simulink model "gm_wlanhdlTimeAndFrequencySynchronization"  (R2025a)
settings: Solver=FixedStepDiscrete  StartTime=0.0  StopTime=stopTime  RelTol=1e-3
InitFcn:
  | wlanFrontEndInit;
undefined symbols (not defined in the file or in its folder): a, b, c, Hd, wlanConfig
libraries: simulink x95, hdlsllib x16, hdlmdlgenlib x12, dspsrcs4 x3, dspsigops x3, dsphdlsigops2 x2, dsphdlfiltering2 x2
(part 5 of 11)

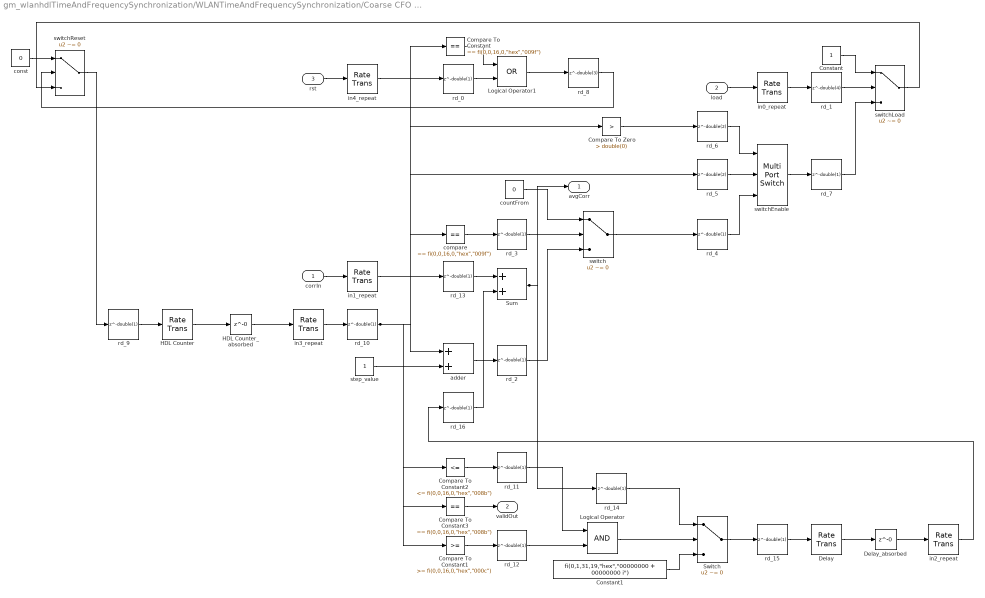
== system gm_wlanhdlTimeAndFrequencySynchronization/WLANTimeAndFrequencySynchronization/Coarse CFO Estimation and Correction/Coarse CFO Estimation/Averager ==
  corrIn : Inport  OutDataTypeStr=fixdt(1, 31, 19)  PortDimensions=1  SampleTime=5e-08
      settings: SignalType=complex
  load : Inport  Port=2  OutDataTypeStr=boolean  PortDimensions=1  SampleTime=5e-08
  rst : Inport  Port=3  OutDataTypeStr=boolean  PortDimensions=1  SampleTime=5e-08
  Compare To Constant : simulink/Logic and Bit Operations/Compare To Constant  relop===  const="fi(0,0,16,0,\"hex\",\"009f\")"  OutDataTypeStr=boolean
  Compare To Constant1 : simulink/Logic and Bit Operations/Compare To Constant  relop=>=  const="fi(0,0,16,0,\"hex\",\"000c\")"  OutDataTypeStr=boolean
  Compare To Constant2 : simulink/Logic and Bit Operations/Compare To Constant  relop=<=  const="fi(0,0,16,0,\"hex\",\"008b\")"  OutDataTypeStr=boolean
  Compare To Constant3 : simulink/Logic and Bit Operations/Compare To Constant  relop===  const="fi(0,0,16,0,\"hex\",\"008b\")"  OutDataTypeStr=boolean
  Compare To Zero : simulink/Logic and Bit Operations/Compare To Constant  relop=>  const=double(0)  OutDataTypeStr=boolean
  Constant : Constant  OutDataTypeStr=uint16  SampleTime=6.25e-09
  Constant1 : Constant  Value="fi(0,1,31,19,\"hex\",\"00000000 + 00000000 i\")"  OutDataTypeStr=fixdt(1, 31, 19)  SampleTime=6.25e-09
  Delay : RateTransition  InitialCondition=double(0)  OutPortSampleTimeOpt=Multiple of input port sample time  OutPortSampleTimeMultiple=8
  Delay_absorbed : Delay  DelayLength=0
  HDL Counter : RateTransition  InitialCondition=double(0)  OutPortSampleTimeOpt=Multiple of input port sample time  OutPortSampleTimeMultiple=8
  HDL Counter_absorbed : Delay  DelayLength=0
  Logical Operator : Logic  AllPortsSameDT=off  OutDataTypeStr=boolean  SampleTime=6.25e-09
  Logical Operator1 : Logic  Operator=OR  AllPortsSameDT=off  OutDataTypeStr=boolean  SampleTime=6.25e-09
  Sum : Sum  OutDataTypeStr=fixdt(1, 31, 19)  AccumDataTypeStr=fixdt(1, 32, 19)  SampleTime=6.25e-09
  Switch : Switch  Criteria=u2 ~= 0  Threshold="fi(0,0,1,0,\"hex\",\"0\")"  OutDataTypeStr=fixdt(1, 31, 19)  SampleTime=6.25e-09  SaturateOnIntegerOverflow=off  InputSameDT=off
  adder : Sum  OutDataTypeStr=uint16  AccumDataTypeStr=uint16  SampleTime=6.25e-09
  compare : simulink/Logic and Bit Operations/Compare To Constant  relop===  const="fi(0,0,16,0,\"hex\",\"009f\")"  OutDataTypeStr=boolean
  const : Constant  Value=0  VectorParams1D=off  OutDataTypeStr=uint16  SampleTime=6.25e-09
  countFrom : Constant  Value=0  VectorParams1D=off  OutDataTypeStr=uint16  SampleTime=6.25e-09
  in0_repeat : RateTransition  Integrity=off  Deterministic=off  OutPortSampleTimeOpt=Multiple of input port sample time  OutPortSampleTimeMultiple=1/8
  in1_repeat : RateTransition  Integrity=off  Deterministic=off  OutPortSampleTimeOpt=Multiple of input port sample time  OutPortSampleTimeMultiple=1/8
  in2_repeat : RateTransition  Integrity=off  Deterministic=off  OutPortSampleTimeOpt=Multiple of input port sample time  OutPortSampleTimeMultiple=1/8
  in3_repeat : RateTransition  Integrity=off  Deterministic=off  OutPortSampleTimeOpt=Multiple of input port sample time  OutPortSampleTimeMultiple=1/8
  in4_repeat : RateTransition  Integrity=off  Deterministic=off  OutPortSampleTimeOpt=Multiple of input port sample time  OutPortSampleTimeMultiple=1/8
  rd_{0,2..4,7,9..16} (13 alike) : Delay  DelayLength=double(1)  InitialCondition=0  SampleTime=6.25e-09
  rd_1 : Delay  DelayLength=double(4)  InitialCondition=0  SampleTime=6.25e-09
  rd_5 : Delay  DelayLength=double(2)  InitialCondition=0  SampleTime=6.25e-09
  rd_6 : Delay  DelayLength=double(2)  InitialCondition=0  SampleTime=6.25e-09
  rd_8 : Delay  DelayLength=double(3)  InitialCondition=0  SampleTime=6.25e-09
  step_value : Constant  VectorParams1D=off  OutDataTypeStr=uint16  SampleTime=6.25e-09
  switch : Switch  Criteria=u2 ~= 0  Threshold="fi(0,0,1,0,\"hex\",\"0\")"  OutDataTypeStr=uint16  SampleTime=6.25e-09  SaturateOnIntegerOverflow=off  InputSameDT=off
  switchEnable : MultiPortSwitch  DataPortOrder=Zero-based contiguous  Inputs=2  DiagnosticForDefault=None  zeroidx=on  OutDataTypeStr=uint16  SampleTime=6.25e-09  SaturateOnIntegerOverflow=off  InputSameDT=off
  switchLoad : Switch  Criteria=u2 ~= 0  Threshold="fi(0,0,1,0,\"hex\",\"0\")"  OutDataTypeStr=uint16  SampleTime=6.25e-09  SaturateOnIntegerOverflow=off  InputSameDT=off
  switchReset : Switch  Criteria=u2 ~= 0  Threshold="fi(0,0,1,0,\"hex\",\"0\")"  OutDataTypeStr=uint16  SampleTime=6.25e-09  SaturateOnIntegerOverflow=off  InputSameDT=off
  avgCorr : Outport  SampleTime=6.25e-09
  validOut : Outport  Port=2  SampleTime=6.25e-09
  wires:
  in2_repeat/1 -> rd_16/1
  Delay/1 -> Delay_absorbed/1
  rd_7/1 -> switchLoad/3
  rd_1/1 -> switchLoad/2
  Constant/1 -> switchLoad/1
  in0_repeat/1 -> rd_1/1
  Switch/1 -> rd_15/1
  rd_4/1 -> switchEnable/3
  rd_5/1 -> switchEnable/2
  load/1 -> in0_repeat/1
  Constant1/1 -> Switch/3
  rd_15/1 -> Delay/1
  rd_6/1 -> switchEnable/1
  Logical Operator/1 -> Switch/2
  switch/1 -> rd_4/1
  Compare To Zero/1 -> rd_6/1
  step_value/1 -> adder/2
  rd_3/1 -> switch/2
  rd_13/1 -> Sum/1
  rd_10/1 -> Compare To Constant3/1, Compare To Constant2/1, adder/1, compare/1, Compare To Constant/1, Compare To Constant1/1, rd_5/1, Compare To Zero/1
  Logical Operator1/1 -> rd_8/1
  Delay_absorbed/1 -> in2_repeat/1
  in3_repeat/1 -> rd_10/1
  adder/1 -> rd_2/1
  in1_repeat/1 -> rd_13/1
  HDL Counter/1 -> HDL Counter_absorbed/1
  rst/1 -> in4_repeat/1
  Compare To Constant2/1 -> rd_11/1
  rd_9/1 -> HDL Counter/1
  HDL Counter_absorbed/1 -> in3_repeat/1
  Sum/1 -> avgCorr/1, rd_14/1
  switchReset/1 -> rd_9/1
  Compare To Constant/1 -> Logical Operator1/1
  corrIn/1 -> in1_repeat/1
  const/1 -> switchReset/1
  compare/1 -> rd_3/1
  rd_16/1 -> Sum/2
  Compare To Constant1/1 -> rd_12/1
  Compare To Constant3/1 -> validOut/1
  switchEnable/1 -> rd_7/1
  rd_14/1 -> Switch/1
  countFrom/1 -> switch/1
  rd_0/1 -> Logical Operator1/2
  rd_2/1 -> switch/3
  switchLoad/1 -> switchReset/3
  rd_11/1 -> Logical Operator/1
  rd_12/1 -> Logical Operator/2
  in4_repeat/1 -> rd_0/1
  rd_8/1 -> switchReset/2

== system gm_wlanhdlTimeAndFrequencySynchronization/WLANTimeAndFrequencySynchronization/Coarse CFO Estimation and Correction/Coarse CFO Estimation/Correlator ==
  dataIn : Inport  OutDataTypeStr=fixdt(1, 16, 12)  PortDimensions=1  SampleTime=5e-08
      settings: SignalType=complex
  lstf_start : Inport  Port=2  OutDataTypeStr=boolean  PortDimensions=1  SampleTime=6.25e-09
  Data Type Conversion : DataTypeConversion  OutDataTypeStr=fixdt(1, 31, 19)  SampleTime=6.25e-09  SaturateOnIntegerOverflow=off  RndMeth=Floor
  Delay1 : Delay  DelayLength=double(2)  InitialCondition=0  SampleTime=5e-08
  Delay2 : Delay  DelayLength=double(16)  InitialCondition=0  SampleTime=5e-08
  Delay3 : Delay  DelayLength=double(2)  InitialCondition=0  SampleTime=5e-08
  Delay4 : Delay  DelayLength=double(15)  InitialCondition=0  SampleTime=5e-08
  Delay41 : RateTransition  InitialCondition=double(0)  OutPortSampleTimeOpt=Multiple of input port sample time  OutPortSampleTimeMultiple=8
  Delay5 : Delay  DelayLength=double(2)  InitialCondition=0  SampleTime=5e-08
  HwModeRegister{,1..9} (10 alike) : Delay  DelayLength=double(1)  InitialCondition=0  SampleTime=6.25e-09
  MultiplyAdd : hdlsllib/HDL Operations/Multiply-Add  Function=c-(a.*b)  datatype=fixdt(1, 33, 24)  RndMeth=Round  DoSatur=off  FMA=off
  MultiplyAdd1 : hdlsllib/HDL Operations/Multiply-Add  Function=c+(a.*b)  datatype=fixdt(1, 33, 24)  RndMeth=Round  DoSatur=off  FMA=off
  MultiplyAdd_out_dtc : DataTypeConversion  OutDataTypeStr=fixdt(1, 32, 24)  RndMeth=Round  SampleTime=6.25e-09  SaturateOnIntegerOverflow=off
  MultiplyAdd_out_dtc1 : DataTypeConversion  OutDataTypeStr=fixdt(1, 32, 24)  RndMeth=Round  SampleTime=6.25e-09  SaturateOnIntegerOverflow=off
  PipelineRegister : Delay  DelayLength=double(1)  InitialCondition=0  SampleTime=6.25e-09
  PipelineRegister1 : Delay  DelayLength=double(1)  InitialCondition=0  SampleTime=6.25e-09
  PipelineRegister2 : Delay  DelayLength=double(2)  InitialCondition=0  SampleTime=6.25e-09
  PipelineRegister3 : Delay  DelayLength=double(2)  InitialCondition=0  SampleTime=6.25e-09
  Product : Product  Inputs=**  OutDataTypeStr=fixdt(1, 32, 24)  RndMeth=Round  SampleTime=6.25e-09
  Product1 : Product  Inputs=**  OutDataTypeStr=fixdt(1, 32, 24)  RndMeth=Round  SampleTime=6.25e-09
  Product_C2ReIm_1 : ComplexToRealImag  SampleTime=6.25e-09
  Product_C2ReIm_2 : ComplexToRealImag  SampleTime=6.25e-09
  Product_ReIm2Complex : RealImagToComplex  SampleTime=6.25e-09
  complexConj : Math  Operator=conj  SignedPower=on  OutDataTypeStr=fixdt(1, 16, 12)  SaturateOnIntegerOverflow=off
  crp_out_delay : Delay  DelayLength=double(1)  InitialCondition=0  SampleTime=6.25e-09
  in1_repeat : RateTransition  Integrity=off  Deterministic=off  OutPortSampleTimeOpt=Multiple of input port sample time  OutPortSampleTimeMultiple=1/8
  in2_repeat : RateTransition  Integrity=off  Deterministic=off  OutPortSampleTimeOpt=Multiple of input port sample time  OutPortSampleTimeMultiple=1/8
  rd_{1,3,6..7} (4 alike) : Delay  DelayLength=double(1)  InitialCondition=0  SampleTime=6.25e-09
  rd_2 : Delay  DelayLength=double(2)  InitialCondition=0  SampleTime=6.25e-09
  rd_4 : Delay  DelayLength=double(2)  InitialCondition=0  SampleTime=6.25e-09
  rd_5 : Delay  DelayLength=double(2)  InitialCondition=0  SampleTime=6.25e-09
  corrOut : Outport  SampleTime=6.25e-09
  load : Outport  Port=2  SampleTime=5e-08
  wires:
  Data Type Conversion/1 -> corrOut/1
  Product_ReIm2Complex/1 -> Data Type Conversion/1
  MultiplyAdd_out_dtc1/1 -> Product_ReIm2Complex/2
  MultiplyAdd_out_dtc/1 -> Product_ReIm2Complex/1
  rd_7/1 -> MultiplyAdd_out_dtc1/1
  rd_6/1 -> MultiplyAdd_out_dtc/1
  MultiplyAdd/1 -> PipelineRegister2/1
  PipelineRegister3/1 -> rd_7/1
  HwModeRegister7/1 -> MultiplyAdd1/1
  HwModeRegister6/1 -> MultiplyAdd/3
  rd_3/1 -> Product_C2ReIm_2/1
  HwModeRegister3/1 -> Product1/2
  PipelineRegister/1 -> HwModeRegister6/1
  Delay3/1 -> in2_repeat/1
  Delay4/1 -> Delay5/1
  HwModeRegister1/1 -> Product/2
  in2_repeat/1 -> rd_3/1
  in1_repeat/1 -> rd_1/1
  Product_C2ReIm_1/2 -> rd_2/1
  complexConj/1 -> Delay3/1
  Delay41/1 -> Delay4/1
  HwModeRegister2/1 -> Product1/1
  Delay1/1 -> in1_repeat/1
  Delay2/1 -> complexConj/1
  PipelineRegister2/1 -> rd_6/1
  HwModeRegister9/1 -> MultiplyAdd1/3
  crp_out_delay/1 -> Delay41/1
  lstf_start/1 -> crp_out_delay/1
  HwModeRegister4/1 -> MultiplyAdd/1
  dataIn/1 -> Delay1/1, Delay2/1
  Product_C2ReIm_1/1 -> HwModeRegister2/1, HwModeRegister/1
  PipelineRegister1/1 -> HwModeRegister9/1
  rd_1/1 -> Product_C2ReIm_1/1
  Product_C2ReIm_2/1 -> HwModeRegister1/1, rd_5/1
  MultiplyAdd1/1 -> PipelineRegister3/1
  rd_4/1 -> HwModeRegister5/1
  HwModeRegister/1 -> Product/1
  rd_5/1 -> HwModeRegister8/1
  Product_C2ReIm_2/2 -> HwModeRegister3/1, rd_4/1
  HwModeRegister5/1 -> MultiplyAdd/2
  Delay5/1 -> load/1
  Product/1 -> PipelineRegister/1
  HwModeRegister8/1 -> MultiplyAdd1/2
  Product1/1 -> PipelineRegister1/1
  rd_2/1 -> HwModeRegister7/1, HwModeRegister4/1

== system gm_wlanhdlTimeAndFrequencySynchronization/WLANTimeAndFrequencySynchronization/Coarse CFO Estimation and Correction/Coarse CFO Estimation/Iteration ==
  xin : Inport  OutDataTypeStr=fixdt(1, 32, 19)  SampleTime=6.25e-09
  yin : Inport  Port=2  OutDataTypeStr=fixdt(1, 32, 19)  SampleTime=6.25e-09
  zin : Inport  Port=3  OutDataTypeStr=fixdt(1, 34, 33)  SampleTime=6.25e-09
  lut_value : Inport  Port=4  OutDataTypeStr=fixdt(0, 31, 33)  SampleTime=6.25e-09
  idx : Inport  Port=5  OutDataTypeStr=fixdt(0, 6, 0)  SampleTime=6.25e-09
  MuxX : Switch  Criteria=u2 ~= 0  Threshold="fi(0,0,1,0,\"hex\",\"0\")"  OutDataTypeStr=fixdt(1, 32, 19)  SampleTime=6.25e-09  SaturateOnIntegerOverflow=off  InputSameDT=off
  MuxY : Switch  Criteria=u2 ~= 0  Threshold="fi(0,0,1,0,\"hex\",\"0\")"  OutDataTypeStr=fixdt(1, 32, 19)  SampleTime=6.25e-09  SaturateOnIntegerOverflow=off  InputSameDT=off
  MuxZ : Switch  Criteria=u2 ~= 0  Threshold="fi(0,0,1,0,\"hex\",\"0\")"  OutDataTypeStr=fixdt(1, 34, 33)  SampleTime=6.25e-09  SaturateOnIntegerOverflow=off  InputSameDT=off
  XAdder : Sum  OutDataTypeStr=fixdt(1, 32, 19)  SampleTime=6.25e-09
  XSubtractor : Sum  Inputs=+-  OutDataTypeStr=fixdt(1, 32, 19)  AccumDataTypeStr=fixdt(1, 32, 19)  SampleTime=6.25e-09
  YAdder : Sum  OutDataTypeStr=fixdt(1, 32, 19)  SampleTime=6.25e-09
  YSub : Sum  Inputs=+-  OutDataTypeStr=fixdt(1, 32, 19)  AccumDataTypeStr=fixdt(1, 32, 19)  SampleTime=6.25e-09
  ZAdder : Sum  OutDataTypeStr=fixdt(1, 34, 33)  SampleTime=6.25e-09
  ZSub : Sum  Inputs=+-  OutDataTypeStr=fixdt(1, 34, 33)  AccumDataTypeStr=fixdt(1, 34, 33)  SampleTime=6.25e-09
  compare : simulink/Logic and Bit Operations/Compare To Constant  relop=<  const=double(0)  OutDataTypeStr=boolean
  dynamic_shift : ArithShift  BitShiftNumberSource=Input port  BitShiftDirection=Right
      settings: InputPortMap=u0,p1
  dynamic_shift1 : ArithShift  BitShiftNumberSource=Input port  BitShiftDirection=Right
      settings: InputPortMap=u0,p1
  rd_{0..8} (9 alike) : Delay  DelayLength=double(1)  InitialCondition=0  SampleTime=6.25e-09
  xout : Outport  OutDataTypeStr=fixdt(1, 32, 19)  SampleTime=6.25e-09
  yout : Outport  Port=2  OutDataTypeStr=fixdt(1, 32, 19)  SampleTime=6.25e-09
  zout : Outport  Port=3  OutDataTypeStr=fixdt(1, 34, 33)  SampleTime=6.25e-09
  wires:
  MuxY/1 -> yout/1
  rd_6/1 -> MuxY/3
  rd_3/1 -> MuxX/2, MuxY/2, MuxZ/2
  rd_4/1 -> MuxX/3
  YSub/1 -> rd_6/1
  ZAdder/1 -> rd_8/1
  xin/1 -> rd_0/1
  MuxZ/1 -> zout/1
  MuxX/1 -> xout/1
  rd_7/1 -> MuxZ/1
  rd_2/1 -> MuxX/1
  yin/1 -> rd_1/1
  XSubtractor/1 -> rd_2/1
  YAdder/1 -> rd_5/1
  rd_1/1 -> compare/1, dynamic_shift1/1, YAdder/1, YSub/1
  idx/1 -> dynamic_shift/2, dynamic_shift1/2
  rd_8/1 -> MuxZ/3
  lut_value/1 -> ZSub/2, ZAdder/2
  rd_5/1 -> MuxY/1
  rd_0/1 -> dynamic_shift/1, XSubtractor/1, XAdder/1
  ZSub/1 -> rd_7/1
  dynamic_shift1/1 -> XSubtractor/2, XAdder/2
  zin/1 -> ZSub/1, ZAdder/1
  compare/1 -> rd_3/1
  dynamic_shift/1 -> YAdder/2, YSub/2
  XAdder/1 -> rd_4/1

== system gm_wlanhdlTimeAndFrequencySynchronization/WLANTimeAndFrequencySynchronization/Coarse CFO Estimation and Correction/Coarse CFO Estimation/Iteration1 ==
  xin : Inport  OutDataTypeStr=fixdt(1, 32, 19)  SampleTime=6.25e-09
  yin : Inport  Port=2  OutDataTypeStr=fixdt(1, 32, 19)  SampleTime=6.25e-09
  zin : Inport  Port=3  OutDataTypeStr=fixdt(1, 34, 33)  SampleTime=6.25e-09
  lut_value : Inport  Port=4  OutDataTypeStr=fixdt(0, 31, 33)  SampleTime=6.25e-09
  idx : Inport  Port=5  OutDataTypeStr=fixdt(0, 6, 0)  SampleTime=6.25e-09
  MuxX : Switch  Criteria=u2 ~= 0  Threshold="fi(0,0,1,0,\"hex\",\"0\")"  OutDataTypeStr=fixdt(1, 32, 19)  SampleTime=6.25e-09  SaturateOnIntegerOverflow=off  InputSameDT=off
  MuxY : Switch  Criteria=u2 ~= 0  Threshold="fi(0,0,1,0,\"hex\",\"0\")"  OutDataTypeStr=fixdt(1, 32, 19)  SampleTime=6.25e-09  SaturateOnIntegerOverflow=off  InputSameDT=off
  MuxZ : Switch  Criteria=u2 ~= 0  Threshold="fi(0,0,1,0,\"hex\",\"0\")"  OutDataTypeStr=fixdt(1, 34, 33)  SampleTime=6.25e-09  SaturateOnIntegerOverflow=off  InputSameDT=off
  XAdder : Sum  OutDataTypeStr=fixdt(1, 32, 19)  SampleTime=6.25e-09
  XSubtractor : Sum  Inputs=+-  OutDataTypeStr=fixdt(1, 32, 19)  AccumDataTypeStr=fixdt(1, 32, 19)  SampleTime=6.25e-09
  YAdder : Sum  OutDataTypeStr=fixdt(1, 32, 19)  SampleTime=6.25e-09
  YSub : Sum  Inputs=+-  OutDataTypeStr=fixdt(1, 32, 19)  AccumDataTypeStr=fixdt(1, 32, 19)  SampleTime=6.25e-09
  ZAdder : Sum  OutDataTypeStr=fixdt(1, 34, 33)  SampleTime=6.25e-09
  ZSub : Sum  Inputs=+-  OutDataTypeStr=fixdt(1, 34, 33)  AccumDataTypeStr=fixdt(1, 34, 33)  SampleTime=6.25e-09
  compare : simulink/Logic and Bit Operations/Compare To Constant  relop=<  const=double(0)  OutDataTypeStr=boolean
  dynamic_shift : ArithShift  BitShiftNumberSource=Input port  BitShiftDirection=Right
      settings: InputPortMap=u0,p1
  dynamic_shift1 : ArithShift  BitShiftNumberSource=Input port  BitShiftDirection=Right
      settings: InputPortMap=u0,p1
  rd_{0..9} (10 alike) : Delay  DelayLength=double(1)  InitialCondition=0  SampleTime=6.25e-09
  xout : Outport  OutDataTypeStr=fixdt(1, 32, 19)  SampleTime=6.25e-09
  yout : Outport  Port=2  OutDataTypeStr=fixdt(1, 32, 19)  SampleTime=6.25e-09
  zout : Outport  Port=3  OutDataTypeStr=fixdt(1, 34, 33)  SampleTime=6.25e-09
  wires:
  rd_3/1 -> MuxX/2, MuxY/2, MuxZ/2
  rd_4/1 -> MuxX/3
  rd_6/1 -> MuxY/3
  MuxZ/1 -> zout/1
  XSubtractor/1 -> rd_2/1
  yin/1 -> rd_1/1
  dynamic_shift/1 -> YAdder/2, YSub/2
  YAdder/1 -> rd_5/1
  rd_8/1 -> MuxZ/1
  XAdder/1 -> rd_4/1
  xin/1 -> rd_0/1
  MuxY/1 -> yout/1
  rd_0/1 -> dynamic_shift/1, XSubtractor/1, XAdder/1
  rd_5/1 -> MuxY/1
  dynamic_shift1/1 -> XSubtractor/2, XAdder/2
  rd_1/1 -> compare/1, dynamic_shift1/1, YAdder/1, YSub/1
  rd_2/1 -> MuxX/1
  zin/1 -> rd_7/1
  idx/1 -> dynamic_shift/2, dynamic_shift1/2
  rd_9/1 -> MuxZ/3
  lut_value/1 -> ZSub/2, ZAdder/2
  MuxX/1 -> xout/1
  ZAdder/1 -> rd_9/1
  rd_7/1 -> ZSub/1, ZAdder/1
  ZSub/1 -> rd_8/1
  YSub/1 -> rd_6/1
  compare/1 -> rd_3/1

== system gm_wlanhdlTimeAndFrequencySynchronization/WLANTimeAndFrequencySynchronization/Coarse CFO Estimation and Correction/Coarse CFO Estimation/Iteration10 ==
  xin : Inport  OutDataTypeStr=fixdt(1, 32, 19)  SampleTime=6.25e-09
  yin : Inport  Port=2  OutDataTypeStr=fixdt(1, 32, 19)  SampleTime=6.25e-09
  zin : Inport  Port=3  OutDataTypeStr=fixdt(1, 34, 33)  SampleTime=6.25e-09
  lut_value : Inport  Port=4  OutDataTypeStr=fixdt(0, 31, 33)  SampleTime=6.25e-09
  idx : Inport  Port=5  OutDataTypeStr=fixdt(0, 6, 0)  SampleTime=6.25e-09
  MuxX : Switch  Criteria=u2 ~= 0  Threshold="fi(0,0,1,0,\"hex\",\"0\")"  OutDataTypeStr=fixdt(1, 32, 19)  SampleTime=6.25e-09  SaturateOnIntegerOverflow=off  InputSameDT=off
  MuxY : Switch  Criteria=u2 ~= 0  Threshold="fi(0,0,1,0,\"hex\",\"0\")"  OutDataTypeStr=fixdt(1, 32, 19)  SampleTime=6.25e-09  SaturateOnIntegerOverflow=off  InputSameDT=off
  MuxZ : Switch  Criteria=u2 ~= 0  Threshold="fi(0,0,1,0,\"hex\",\"0\")"  OutDataTypeStr=fixdt(1, 34, 33)  SampleTime=6.25e-09  SaturateOnIntegerOverflow=off  InputSameDT=off
  XAdder : Sum  OutDataTypeStr=fixdt(1, 32, 19)  SampleTime=6.25e-09
  XSubtractor : Sum  Inputs=+-  OutDataTypeStr=fixdt(1, 32, 19)  AccumDataTypeStr=fixdt(1, 32, 19)  SampleTime=6.25e-09
  YAdder : Sum  OutDataTypeStr=fixdt(1, 32, 19)  SampleTime=6.25e-09
  YSub : Sum  Inputs=+-  OutDataTypeStr=fixdt(1, 32, 19)  AccumDataTypeStr=fixdt(1, 32, 19)  SampleTime=6.25e-09
  ZAdder : Sum  OutDataTypeStr=fixdt(1, 34, 33)  SampleTime=6.25e-09
  ZSub : Sum  Inputs=+-  OutDataTypeStr=fixdt(1, 34, 33)  AccumDataTypeStr=fixdt(1, 34, 33)  SampleTime=6.25e-09
  compare : simulink/Logic and Bit Operations/Compare To Constant  relop=<  const=double(0)  OutDataTypeStr=boolean
  dynamic_shift : ArithShift  BitShiftNumberSource=Input port  BitShiftDirection=Right
      settings: InputPortMap=u0,p1
  dynamic_shift1 : ArithShift  BitShiftNumberSource=Input port  BitShiftDirection=Right
      settings: InputPortMap=u0,p1
  rd_{0..9} (10 alike) : Delay  DelayLength=double(1)  InitialCondition=0  SampleTime=6.25e-09
  xout : Outport  OutDataTypeStr=fixdt(1, 32, 19)  SampleTime=6.25e-09
  yout : Outport  Port=2  OutDataTypeStr=fixdt(1, 32, 19)  SampleTime=6.25e-09
  zout : Outport  Port=3  OutDataTypeStr=fixdt(1, 34, 33)  SampleTime=6.25e-09
  wires:
  MuxY/1 -> yout/1
  MuxX/1 -> xout/1
  rd_5/1 -> MuxY/1
  rd_3/1 -> MuxX/2, MuxY/2, MuxZ/2
  rd_8/1 -> MuxZ/1
  rd_4/1 -> MuxX/3
  YSub/1 -> rd_6/1
  xin/1 -> rd_0/1
  MuxZ/1 -> zout/1
  rd_6/1 -> MuxY/3
  ZAdder/1 -> rd_9/1
  yin/1 -> rd_1/1
  rd_0/1 -> dynamic_shift/1, XAdder/1, XSubtractor/1
  zin/1 -> rd_7/1
  rd_2/1 -> MuxX/1
  ZSub/1 -> rd_8/1
  idx/1 -> dynamic_shift1/2, dynamic_shift/2
  rd_1/1 -> compare/1, dynamic_shift1/1, YAdder/1, YSub/1
  dynamic_shift1/1 -> XAdder/2, XSubtractor/2
  rd_7/1 -> ZSub/1, ZAdder/1
  YAdder/1 -> rd_5/1
  lut_value/1 -> ZAdder/2, ZSub/2
  dynamic_shift/1 -> YSub/2, YAdder/2
  XSubtractor/1 -> rd_2/1
  compare/1 -> rd_3/1
  rd_9/1 -> MuxZ/3
  XAdder/1 -> rd_4/1

== system gm_wlanhdlTimeAndFrequencySynchronization/WLANTimeAndFrequencySynchronization/Coarse CFO Estimation and Correction/Coarse CFO Estimation/Iteration11 ==
  xin : Inport  OutDataTypeStr=fixdt(1, 32, 19)  SampleTime=6.25e-09
  yin : Inport  Port=2  OutDataTypeStr=fixdt(1, 32, 19)  SampleTime=6.25e-09
  zin : Inport  Port=3  OutDataTypeStr=fixdt(1, 34, 33)  SampleTime=6.25e-09
  lut_value : Inport  Port=4  OutDataTypeStr=fixdt(0, 31, 33)  SampleTime=6.25e-09
  idx : Inport  Port=5  OutDataTypeStr=fixdt(0, 6, 0)  SampleTime=6.25e-09
  MuxX : Switch  Criteria=u2 ~= 0  Threshold="fi(0,0,1,0,\"hex\",\"0\")"  OutDataTypeStr=fixdt(1, 32, 19)  SampleTime=6.25e-09  SaturateOnIntegerOverflow=off  InputSameDT=off
  MuxY : Switch  Criteria=u2 ~= 0  Threshold="fi(0,0,1,0,\"hex\",\"0\")"  OutDataTypeStr=fixdt(1, 32, 19)  SampleTime=6.25e-09  SaturateOnIntegerOverflow=off  InputSameDT=off
  MuxZ : Switch  Criteria=u2 ~= 0  Threshold="fi(0,0,1,0,\"hex\",\"0\")"  OutDataTypeStr=fixdt(1, 34, 33)  SampleTime=6.25e-09  SaturateOnIntegerOverflow=off  InputSameDT=off
  XAdder : Sum  OutDataTypeStr=fixdt(1, 32, 19)  SampleTime=6.25e-09
  XSubtractor : Sum  Inputs=+-  OutDataTypeStr=fixdt(1, 32, 19)  AccumDataTypeStr=fixdt(1, 32, 19)  SampleTime=6.25e-09
  YAdder : Sum  OutDataTypeStr=fixdt(1, 32, 19)  SampleTime=6.25e-09
  YSub : Sum  Inputs=+-  OutDataTypeStr=fixdt(1, 32, 19)  AccumDataTypeStr=fixdt(1, 32, 19)  SampleTime=6.25e-09
  ZAdder : Sum  OutDataTypeStr=fixdt(1, 34, 33)  SampleTime=6.25e-09
  ZSub : Sum  Inputs=+-  OutDataTypeStr=fixdt(1, 34, 33)  AccumDataTypeStr=fixdt(1, 34, 33)  SampleTime=6.25e-09
  compare : simulink/Logic and Bit Operations/Compare To Constant  relop=<  const=double(0)  OutDataTypeStr=boolean
  dynamic_shift : ArithShift  BitShiftNumberSource=Input port  BitShiftDirection=Right
      settings: InputPortMap=u0,p1
  dynamic_shift1 : ArithShift  BitShiftNumberSource=Input port  BitShiftDirection=Right
      settings: InputPortMap=u0,p1
  rd_{0..9} (10 alike) : Delay  DelayLength=double(1)  InitialCondition=0  SampleTime=6.25e-09
  xout : Outport  OutDataTypeStr=fixdt(1, 32, 19)  SampleTime=6.25e-09
  yout : Outport  Port=2  OutDataTypeStr=fixdt(1, 32, 19)  SampleTime=6.25e-09
  zout : Outport  Port=3  OutDataTypeStr=fixdt(1, 34, 33)  SampleTime=6.25e-09
  wires:
  rd_9/1 -> MuxZ/3
  rd_3/1 -> MuxX/2, MuxY/2, MuxZ/2
  XAdder/1 -> rd_4/1
  MuxX/1 -> xout/1
  XSubtractor/1 -> rd_2/1
  rd_8/1 -> MuxZ/1
  ZAdder/1 -> rd_9/1
  yin/1 -> rd_1/1
  MuxZ/1 -> zout/1
  YSub/1 -> rd_6/1
  MuxY/1 -> yout/1
  ZSub/1 -> rd_8/1
  idx/1 -> dynamic_shift/2, dynamic_shift1/2
  dynamic_shift1/1 -> XSubtractor/2, XAdder/2
  zin/1 -> rd_7/1
  dynamic_shift/1 -> YAdder/2, YSub/2
  rd_0/1 -> dynamic_shift/1, XSubtractor/1, XAdder/1
  rd_6/1 -> MuxY/3
  rd_7/1 -> ZSub/1, ZAdder/1
  compare/1 -> rd_3/1
  rd_4/1 -> MuxX/3
  rd_5/1 -> MuxY/1
  rd_1/1 -> compare/1, dynamic_shift1/1, YAdder/1, YSub/1
  lut_value/1 -> ZSub/2, ZAdder/2
  rd_2/1 -> MuxX/1
  xin/1 -> rd_0/1
  YAdder/1 -> rd_5/1

== system gm_wlanhdlTimeAndFrequencySynchronization/WLANTimeAndFrequencySynchronization/Coarse CFO Estimation and Correction/Coarse CFO Estimation/Iteration12 ==
  xin : Inport  OutDataTypeStr=fixdt(1, 32, 19)  SampleTime=6.25e-09
  yin : Inport  Port=2  OutDataTypeStr=fixdt(1, 32, 19)  SampleTime=6.25e-09
  zin : Inport  Port=3  OutDataTypeStr=fixdt(1, 34, 33)  SampleTime=6.25e-09
  lut_value : Inport  Port=4  OutDataTypeStr=fixdt(0, 31, 33)  SampleTime=6.25e-09
  idx : Inport  Port=5  OutDataTypeStr=fixdt(0, 6, 0)  SampleTime=6.25e-09
  MuxX : Switch  Criteria=u2 ~= 0  Threshold="fi(0,0,1,0,\"hex\",\"0\")"  OutDataTypeStr=fixdt(1, 32, 19)  SampleTime=6.25e-09  SaturateOnIntegerOverflow=off  InputSameDT=off
  MuxY : Switch  Criteria=u2 ~= 0  Threshold="fi(0,0,1,0,\"hex\",\"0\")"  OutDataTypeStr=fixdt(1, 32, 19)  SampleTime=6.25e-09  SaturateOnIntegerOverflow=off  InputSameDT=off
  MuxZ : Switch  Criteria=u2 ~= 0  Threshold="fi(0,0,1,0,\"hex\",\"0\")"  OutDataTypeStr=fixdt(1, 34, 33)  SampleTime=6.25e-09  SaturateOnIntegerOverflow=off  InputSameDT=off
  XAdder : Sum  OutDataTypeStr=fixdt(1, 32, 19)  SampleTime=6.25e-09
  XSubtractor : Sum  Inputs=+-  OutDataTypeStr=fixdt(1, 32, 19)  AccumDataTypeStr=fixdt(1, 32, 19)  SampleTime=6.25e-09
  YAdder : Sum  OutDataTypeStr=fixdt(1, 32, 19)  SampleTime=6.25e-09
  YSub : Sum  Inputs=+-  OutDataTypeStr=fixdt(1, 32, 19)  AccumDataTypeStr=fixdt(1, 32, 19)  SampleTime=6.25e-09
  ZAdder : Sum  OutDataTypeStr=fixdt(1, 34, 33)  SampleTime=6.25e-09
  ZSub : Sum  Inputs=+-  OutDataTypeStr=fixdt(1, 34, 33)  AccumDataTypeStr=fixdt(1, 34, 33)  SampleTime=6.25e-09
  compare : simulink/Logic and Bit Operations/Compare To Constant  relop=<  const=double(0)  OutDataTypeStr=boolean
  dynamic_shift : ArithShift  BitShiftNumberSource=Input port  BitShiftDirection=Right
      settings: InputPortMap=u0,p1
  dynamic_shift1 : ArithShift  BitShiftNumberSource=Input port  BitShiftDirection=Right
      settings: InputPortMap=u0,p1
  rd_{0..9} (10 alike) : Delay  DelayLength=double(1)  InitialCondition=0  SampleTime=6.25e-09
  xout : Outport  OutDataTypeStr=fixdt(1, 32, 19)  SampleTime=6.25e-09
  yout : Outport  Port=2  OutDataTypeStr=fixdt(1, 32, 19)  SampleTime=6.25e-09
  zout : Outport  Port=3  OutDataTypeStr=fixdt(1, 34, 33)  SampleTime=6.25e-09
  wires:
  MuxX/1 -> xout/1
  rd_3/1 -> MuxX/2, MuxY/2, MuxZ/2
  rd_8/1 -> MuxZ/1
  rd_6/1 -> MuxY/3
  XAdder/1 -> rd_4/1
  rd_2/1 -> MuxX/1
  XSubtractor/1 -> rd_2/1
  ZAdder/1 -> rd_9/1
  ZSub/1 -> rd_8/1
  rd_4/1 -> MuxX/3
  yin/1 -> rd_1/1
  xin/1 -> rd_0/1
  rd_5/1 -> MuxY/1
  rd_1/1 -> compare/1, dynamic_shift1/1, YAdder/1, YSub/1
  zin/1 -> rd_7/1
  lut_value/1 -> ZAdder/2, ZSub/2
  MuxZ/1 -> zout/1
  rd_9/1 -> MuxZ/3
  idx/1 -> dynamic_shift1/2, dynamic_shift/2
  MuxY/1 -> yout/1
  rd_7/1 -> ZSub/1, ZAdder/1
  compare/1 -> rd_3/1
  rd_0/1 -> dynamic_shift/1, XSubtractor/1, XAdder/1
  dynamic_shift/1 -> YSub/2, YAdder/2
  YAdder/1 -> rd_5/1
  dynamic_shift1/1 -> XAdder/2, XSubtractor/2
  YSub/1 -> rd_6/1

== system gm_wlanhdlTimeAndFrequencySynchronization/WLANTimeAndFrequencySynchronization/Coarse CFO Estimation and Correction/Coarse CFO Estimation/Iteration13 ==
  xin : Inport  OutDataTypeStr=fixdt(1, 32, 19)  SampleTime=6.25e-09
  yin : Inport  Port=2  OutDataTypeStr=fixdt(1, 32, 19)  SampleTime=6.25e-09
  zin : Inport  Port=3  OutDataTypeStr=fixdt(1, 34, 33)  SampleTime=6.25e-09
  lut_value : Inport  Port=4  OutDataTypeStr=fixdt(0, 31, 33)  SampleTime=6.25e-09
  idx : Inport  Port=5  OutDataTypeStr=fixdt(0, 6, 0)  SampleTime=6.25e-09
  MuxX : Switch  Criteria=u2 ~= 0  Threshold="fi(0,0,1,0,\"hex\",\"0\")"  OutDataTypeStr=fixdt(1, 32, 19)  SampleTime=6.25e-09  SaturateOnIntegerOverflow=off  InputSameDT=off
  MuxY : Switch  Criteria=u2 ~= 0  Threshold="fi(0,0,1,0,\"hex\",\"0\")"  OutDataTypeStr=fixdt(1, 32, 19)  SampleTime=6.25e-09  SaturateOnIntegerOverflow=off  InputSameDT=off
  MuxZ : Switch  Criteria=u2 ~= 0  Threshold="fi(0,0,1,0,\"hex\",\"0\")"  OutDataTypeStr=fixdt(1, 34, 33)  SampleTime=6.25e-09  SaturateOnIntegerOverflow=off  InputSameDT=off
  XAdder : Sum  OutDataTypeStr=fixdt(1, 32, 19)  SampleTime=6.25e-09
  XSubtractor : Sum  Inputs=+-  OutDataTypeStr=fixdt(1, 32, 19)  AccumDataTypeStr=fixdt(1, 32, 19)  SampleTime=6.25e-09
  YAdder : Sum  OutDataTypeStr=fixdt(1, 32, 19)  SampleTime=6.25e-09
  YSub : Sum  Inputs=+-  OutDataTypeStr=fixdt(1, 32, 19)  AccumDataTypeStr=fixdt(1, 32, 19)  SampleTime=6.25e-09
  ZAdder : Sum  OutDataTypeStr=fixdt(1, 34, 33)  SampleTime=6.25e-09
  ZSub : Sum  Inputs=+-  OutDataTypeStr=fixdt(1, 34, 33)  AccumDataTypeStr=fixdt(1, 34, 33)  SampleTime=6.25e-09
  compare : simulink/Logic and Bit Operations/Compare To Constant  relop=<  const=double(0)  OutDataTypeStr=boolean
  dynamic_shift : ArithShift  BitShiftNumberSource=Input port  BitShiftDirection=Right
      settings: InputPortMap=u0,p1
  dynamic_shift1 : ArithShift  BitShiftNumberSource=Input port  BitShiftDirection=Right
      settings: InputPortMap=u0,p1
  rd_{0..9} (10 alike) : Delay  DelayLength=double(1)  InitialCondition=0  SampleTime=6.25e-09
  xout : Outport  OutDataTypeStr=fixdt(1, 32, 19)  SampleTime=6.25e-09
  yout : Outport  Port=2  OutDataTypeStr=fixdt(1, 32, 19)  SampleTime=6.25e-09
  zout : Outport  Port=3  OutDataTypeStr=fixdt(1, 34, 33)  SampleTime=6.25e-09
  wires:
  rd_4/1 -> MuxX/3
  rd_2/1 -> MuxX/1
  rd_8/1 -> MuxZ/1
  XAdder/1 -> rd_4/1
  XSubtractor/1 -> rd_2/1
  ZAdder/1 -> rd_9/1
  rd_6/1 -> MuxY/3
  ZSub/1 -> rd_8/1
  dynamic_shift/1 -> YAdder/2, YSub/2
  xin/1 -> rd_0/1
  idx/1 -> dynamic_shift/2, dynamic_shift1/2
  YSub/1 -> rd_6/1
  rd_3/1 -> MuxX/2, MuxY/2, MuxZ/2
  yin/1 -> rd_1/1
  rd_1/1 -> compare/1, dynamic_shift1/1, YAdder/1, YSub/1
  zin/1 -> rd_7/1
  MuxZ/1 -> zout/1
  rd_9/1 -> MuxZ/3
  compare/1 -> rd_3/1
  rd_5/1 -> MuxY/1
  rd_0/1 -> dynamic_shift/1, XSubtractor/1, XAdder/1
  rd_7/1 -> ZSub/1, ZAdder/1
  lut_value/1 -> ZSub/2, ZAdder/2
  MuxY/1 -> yout/1
  dynamic_shift1/1 -> XSubtractor/2, XAdder/2
  MuxX/1 -> xout/1
  YAdder/1 -> rd_5/1

== system gm_wlanhdlTimeAndFrequencySynchronization/WLANTimeAndFrequencySynchronization/Coarse CFO Estimation and Correction/Coarse CFO Estimation/Iteration14 ==
  xin : Inport  OutDataTypeStr=fixdt(1, 32, 19)  SampleTime=6.25e-09
  yin : Inport  Port=2  OutDataTypeStr=fixdt(1, 32, 19)  SampleTime=6.25e-09
  zin : Inport  Port=3  OutDataTypeStr=fixdt(1, 34, 33)  SampleTime=6.25e-09
  lut_value : Inport  Port=4  OutDataTypeStr=fixdt(0, 31, 33)  SampleTime=6.25e-09
  idx : Inport  Port=5  OutDataTypeStr=fixdt(0, 6, 0)  SampleTime=6.25e-09
  MuxX : Switch  Criteria=u2 ~= 0  Threshold="fi(0,0,1,0,\"hex\",\"0\")"  OutDataTypeStr=fixdt(1, 32, 19)  SampleTime=6.25e-09  SaturateOnIntegerOverflow=off  InputSameDT=off
  MuxY : Switch  Criteria=u2 ~= 0  Threshold="fi(0,0,1,0,\"hex\",\"0\")"  OutDataTypeStr=fixdt(1, 32, 19)  SampleTime=6.25e-09  SaturateOnIntegerOverflow=off  InputSameDT=off
  MuxZ : Switch  Criteria=u2 ~= 0  Threshold="fi(0,0,1,0,\"hex\",\"0\")"  OutDataTypeStr=fixdt(1, 34, 33)  SampleTime=6.25e-09  SaturateOnIntegerOverflow=off  InputSameDT=off
  XAdder : Sum  OutDataTypeStr=fixdt(1, 32, 19)  SampleTime=6.25e-09
  XSubtractor : Sum  Inputs=+-  OutDataTypeStr=fixdt(1, 32, 19)  AccumDataTypeStr=fixdt(1, 32, 19)  SampleTime=6.25e-09
  YAdder : Sum  OutDataTypeStr=fixdt(1, 32, 19)  SampleTime=6.25e-09
  YSub : Sum  Inputs=+-  OutDataTypeStr=fixdt(1, 32, 19)  AccumDataTypeStr=fixdt(1, 32, 19)  SampleTime=6.25e-09
  ZAdder : Sum  OutDataTypeStr=fixdt(1, 34, 33)  SampleTime=6.25e-09
  ZSub : Sum  Inputs=+-  OutDataTypeStr=fixdt(1, 34, 33)  AccumDataTypeStr=fixdt(1, 34, 33)  SampleTime=6.25e-09
  compare : simulink/Logic and Bit Operations/Compare To Constant  relop=<  const=double(0)  OutDataTypeStr=boolean
  dynamic_shift : ArithShift  BitShiftNumberSource=Input port  BitShiftDirection=Right
      settings: InputPortMap=u0,p1
  dynamic_shift1 : ArithShift  BitShiftNumberSource=Input port  BitShiftDirection=Right
      settings: InputPortMap=u0,p1
  rd_{0..9} (10 alike) : Delay  DelayLength=double(1)  InitialCondition=0  SampleTime=6.25e-09
  xout : Outport  OutDataTypeStr=fixdt(1, 32, 19)  SampleTime=6.25e-09
  yout : Outport  Port=2  OutDataTypeStr=fixdt(1, 32, 19)  SampleTime=6.25e-09
  zout : Outport  Port=3  OutDataTypeStr=fixdt(1, 34, 33)  SampleTime=6.25e-09
  wires:
  rd_4/1 -> MuxX/3
  rd_9/1 -> MuxZ/3
  rd_6/1 -> MuxY/3
  XAdder/1 -> rd_4/1
  XSubtractor/1 -> rd_2/1
  rd_2/1 -> MuxX/1
  rd_3/1 -> MuxX/2, MuxY/2, MuxZ/2
  ZSub/1 -> rd_8/1
  MuxX/1 -> xout/1
  MuxZ/1 -> zout/1
  idx/1 -> dynamic_shift1/2, dynamic_shift/2
  xin/1 -> rd_0/1
  rd_1/1 -> compare/1, dynamic_shift1/1, YAdder/1, YSub/1
  zin/1 -> rd_7/1
  MuxY/1 -> yout/1
  YSub/1 -> rd_6/1
  rd_0/1 -> dynamic_shift/1, XSubtractor/1, XAdder/1
  lut_value/1 -> ZAdder/2, ZSub/2
  dynamic_shift/1 -> YSub/2, YAdder/2
  rd_8/1 -> MuxZ/1
  rd_7/1 -> ZSub/1, ZAdder/1
  yin/1 -> rd_1/1
  dynamic_shift1/1 -> XAdder/2, XSubtractor/2
  rd_5/1 -> MuxY/1
  ZAdder/1 -> rd_9/1
  compare/1 -> rd_3/1
  YAdder/1 -> rd_5/1

== system gm_wlanhdlTimeAndFrequencySynchronization/WLANTimeAndFrequencySynchronization/Coarse CFO Estimation and Correction/Coarse CFO Estimation/Iteration15 ==
  xin : Inport  OutDataTypeStr=fixdt(1, 32, 19)  SampleTime=6.25e-09
  yin : Inport  Port=2  OutDataTypeStr=fixdt(1, 32, 19)  SampleTime=6.25e-09
  zin : Inport  Port=3  OutDataTypeStr=fixdt(1, 34, 33)  SampleTime=6.25e-09
  lut_value : Inport  Port=4  OutDataTypeStr=fixdt(0, 31, 33)  SampleTime=6.25e-09
  idx : Inport  Port=5  OutDataTypeStr=fixdt(0, 6, 0)  SampleTime=6.25e-09
  MuxX : Switch  Criteria=u2 ~= 0  Threshold="fi(0,0,1,0,\"hex\",\"0\")"  OutDataTypeStr=fixdt(1, 32, 19)  SampleTime=6.25e-09  SaturateOnIntegerOverflow=off  InputSameDT=off
  MuxY : Switch  Criteria=u2 ~= 0  Threshold="fi(0,0,1,0,\"hex\",\"0\")"  OutDataTypeStr=fixdt(1, 32, 19)  SampleTime=6.25e-09  SaturateOnIntegerOverflow=off  InputSameDT=off
  MuxZ : Switch  Criteria=u2 ~= 0  Threshold="fi(0,0,1,0,\"hex\",\"0\")"  OutDataTypeStr=fixdt(1, 34, 33)  SampleTime=6.25e-09  SaturateOnIntegerOverflow=off  InputSameDT=off
  XAdder : Sum  OutDataTypeStr=fixdt(1, 32, 19)  SampleTime=6.25e-09
  XSubtractor : Sum  Inputs=+-  OutDataTypeStr=fixdt(1, 32, 19)  AccumDataTypeStr=fixdt(1, 32, 19)  SampleTime=6.25e-09
  YAdder : Sum  OutDataTypeStr=fixdt(1, 32, 19)  SampleTime=6.25e-09
  YSub : Sum  Inputs=+-  OutDataTypeStr=fixdt(1, 32, 19)  AccumDataTypeStr=fixdt(1, 32, 19)  SampleTime=6.25e-09
  ZAdder : Sum  OutDataTypeStr=fixdt(1, 34, 33)  SampleTime=6.25e-09
  ZSub : Sum  Inputs=+-  OutDataTypeStr=fixdt(1, 34, 33)  AccumDataTypeStr=fixdt(1, 34, 33)  SampleTime=6.25e-09
  compare : simulink/Logic and Bit Operations/Compare To Constant  relop=<  const=double(0)  OutDataTypeStr=boolean
  dynamic_shift : ArithShift  BitShiftNumberSource=Input port  BitShiftDirection=Right
      settings: InputPortMap=u0,p1
  dynamic_shift1 : ArithShift  BitShiftNumberSource=Input port  BitShiftDirection=Right
      settings: InputPortMap=u0,p1
  rd_{0..9} (10 alike) : Delay  DelayLength=double(1)  InitialCondition=0  SampleTime=6.25e-09
  xout : Outport  OutDataTypeStr=fixdt(1, 32, 19)  SampleTime=6.25e-09
  yout : Outport  Port=2  OutDataTypeStr=fixdt(1, 32, 19)  SampleTime=6.25e-09
  zout : Outport  Port=3  OutDataTypeStr=fixdt(1, 34, 33)  SampleTime=6.25e-09
  wires:
  rd_4/1 -> MuxX/3
  rd_2/1 -> MuxX/1
  rd_9/1 -> MuxZ/3
  rd_3/1 -> MuxX/2, MuxY/2, MuxZ/2
  rd_8/1 -> MuxZ/1
  rd_6/1 -> MuxY/3
  rd_5/1 -> MuxY/1
  ZSub/1 -> rd_8/1
  MuxZ/1 -> zout/1
  xin/1 -> rd_0/1
  lut_value/1 -> ZSub/2, ZAdder/2
  rd_1/1 -> compare/1, dynamic_shift1/1, YAdder/1, YSub/1
  MuxY/1 -> yout/1
  ZAdder/1 -> rd_9/1
  zin/1 -> rd_7/1
  rd_0/1 -> dynamic_shift/1, XSubtractor/1, XAdder/1
  rd_7/1 -> ZSub/1, ZAdder/1
  yin/1 -> rd_1/1
  idx/1 -> dynamic_shift/2, dynamic_shift1/2
  dynamic_shift/1 -> YAdder/2, YSub/2
  MuxX/1 -> xout/1
  XAdder/1 -> rd_4/1
  compare/1 -> rd_3/1
  dynamic_shift1/1 -> XSubtractor/2, XAdder/2
  XSubtractor/1 -> rd_2/1
  YSub/1 -> rd_6/1
  YAdder/1 -> rd_5/1

== system gm_wlanhdlTimeAndFrequencySynchronization/WLANTimeAndFrequencySynchronization/Coarse CFO Estimation and Correction/Coarse CFO Estimation/Iteration16 ==
  xin : Inport  OutDataTypeStr=fixdt(1, 32, 19)  SampleTime=6.25e-09
  yin : Inport  Port=2  OutDataTypeStr=fixdt(1, 32, 19)  SampleTime=6.25e-09
  zin : Inport  Port=3  OutDataTypeStr=fixdt(1, 34, 33)  SampleTime=6.25e-09
  lut_value : Inport  Port=4  OutDataTypeStr=fixdt(0, 31, 33)  SampleTime=6.25e-09
  idx : Inport  Port=5  OutDataTypeStr=fixdt(0, 6, 0)  SampleTime=6.25e-09
  MuxX : Switch  Criteria=u2 ~= 0  Threshold="fi(0,0,1,0,\"hex\",\"0\")"  OutDataTypeStr=fixdt(1, 32, 19)  SampleTime=6.25e-09  SaturateOnIntegerOverflow=off  InputSameDT=off
  MuxY : Switch  Criteria=u2 ~= 0  Threshold="fi(0,0,1,0,\"hex\",\"0\")"  OutDataTypeStr=fixdt(1, 32, 19)  SampleTime=6.25e-09  SaturateOnIntegerOverflow=off  InputSameDT=off
  MuxZ : Switch  Criteria=u2 ~= 0  Threshold="fi(0,0,1,0,\"hex\",\"0\")"  OutDataTypeStr=fixdt(1, 34, 33)  SampleTime=6.25e-09  SaturateOnIntegerOverflow=off  InputSameDT=off
  XAdder : Sum  OutDataTypeStr=fixdt(1, 32, 19)  SampleTime=6.25e-09
  XSubtractor : Sum  Inputs=+-  OutDataTypeStr=fixdt(1, 32, 19)  AccumDataTypeStr=fixdt(1, 32, 19)  SampleTime=6.25e-09
  YAdder : Sum  OutDataTypeStr=fixdt(1, 32, 19)  SampleTime=6.25e-09
  YSub : Sum  Inputs=+-  OutDataTypeStr=fixdt(1, 32, 19)  AccumDataTypeStr=fixdt(1, 32, 19)  SampleTime=6.25e-09
  ZAdder : Sum  OutDataTypeStr=fixdt(1, 34, 33)  SampleTime=6.25e-09
  ZSub : Sum  Inputs=+-  OutDataTypeStr=fixdt(1, 34, 33)  AccumDataTypeStr=fixdt(1, 34, 33)  SampleTime=6.25e-09
  compare : simulink/Logic and Bit Operations/Compare To Constant  relop=<  const=double(0)  OutDataTypeStr=boolean
  dynamic_shift : ArithShift  BitShiftNumberSource=Input port  BitShiftDirection=Right
      settings: InputPortMap=u0,p1
  dynamic_shift1 : ArithShift  BitShiftNumberSource=Input port  BitShiftDirection=Right
      settings: InputPortMap=u0,p1
  rd_{0..9} (10 alike) : Delay  DelayLength=double(1)  InitialCondition=0  SampleTime=6.25e-09
  xout : Outport  OutDataTypeStr=fixdt(1, 32, 19)  SampleTime=6.25e-09
  yout : Outport  Port=2  OutDataTypeStr=fixdt(1, 32, 19)  SampleTime=6.25e-09
  zout : Outport  Port=3  OutDataTypeStr=fixdt(1, 34, 33)  SampleTime=6.25e-09
  wires:
  MuxY/1 -> yout/1
  MuxZ/1 -> zout/1
  rd_5/1 -> MuxY/1
  rd_3/1 -> MuxX/2, MuxY/2, MuxZ/2
  YSub/1 -> rd_6/1
  YAdder/1 -> rd_5/1
  ZAdder/1 -> rd_9/1
  ZSub/1 -> rd_8/1
  rd_8/1 -> MuxZ/1
  xin/1 -> rd_0/1
  rd_6/1 -> MuxY/3
  compare/1 -> rd_3/1
  rd_0/1 -> dynamic_shift/1, XSubtractor/1, XAdder/1
  yin/1 -> rd_1/1
  zin/1 -> rd_7/1
  MuxX/1 -> xout/1
  rd_1/1 -> compare/1, dynamic_shift1/1, YAdder/1, YSub/1
  rd_9/1 -> MuxZ/3
  dynamic_shift1/1 -> XAdder/2, XSubtractor/2
  lut_value/1 -> ZAdder/2, ZSub/2
  XSubtractor/1 -> rd_2/1
  rd_7/1 -> ZSub/1, ZAdder/1
  rd_4/1 -> MuxX/3
  rd_2/1 -> MuxX/1
  dynamic_shift/1 -> YSub/2, YAdder/2
  idx/1 -> dynamic_shift1/2, dynamic_shift/2
  XAdder/1 -> rd_4/1

== system gm_wlanhdlTimeAndFrequencySynchronization/WLANTimeAndFrequencySynchronization/Coarse CFO Estimation and Correction/Coarse CFO Estimation/Iteration17 ==
  xin : Inport  OutDataTypeStr=fixdt(1, 32, 19)  SampleTime=6.25e-09
  yin : Inport  Port=2  OutDataTypeStr=fixdt(1, 32, 19)  SampleTime=6.25e-09
  zin : Inport  Port=3  OutDataTypeStr=fixdt(1, 34, 33)  SampleTime=6.25e-09
  lut_value : Inport  Port=4  OutDataTypeStr=fixdt(0, 31, 33)  SampleTime=6.25e-09
  idx : Inport  Port=5  OutDataTypeStr=fixdt(0, 6, 0)  SampleTime=6.25e-09
  MuxX : Switch  Criteria=u2 ~= 0  Threshold="fi(0,0,1,0,\"hex\",\"0\")"  OutDataTypeStr=fixdt(1, 32, 19)  SampleTime=6.25e-09  SaturateOnIntegerOverflow=off  InputSameDT=off
  MuxY : Switch  Criteria=u2 ~= 0  Threshold="fi(0,0,1,0,\"hex\",\"0\")"  OutDataTypeStr=fixdt(1, 32, 19)  SampleTime=6.25e-09  SaturateOnIntegerOverflow=off  InputSameDT=off
  MuxZ : Switch  Criteria=u2 ~= 0  Threshold="fi(0,0,1,0,\"hex\",\"0\")"  OutDataTypeStr=fixdt(1, 34, 33)  SampleTime=6.25e-09  SaturateOnIntegerOverflow=off  InputSameDT=off
  XAdder : Sum  OutDataTypeStr=fixdt(1, 32, 19)  SampleTime=6.25e-09
  XSubtractor : Sum  Inputs=+-  OutDataTypeStr=fixdt(1, 32, 19)  AccumDataTypeStr=fixdt(1, 32, 19)  SampleTime=6.25e-09
  YAdder : Sum  OutDataTypeStr=fixdt(1, 32, 19)  SampleTime=6.25e-09
  YSub : Sum  Inputs=+-  OutDataTypeStr=fixdt(1, 32, 19)  AccumDataTypeStr=fixdt(1, 32, 19)  SampleTime=6.25e-09
  ZAdder : Sum  OutDataTypeStr=fixdt(1, 34, 33)  SampleTime=6.25e-09
  ZSub : Sum  Inputs=+-  OutDataTypeStr=fixdt(1, 34, 33)  AccumDataTypeStr=fixdt(1, 34, 33)  SampleTime=6.25e-09
  compare : simulink/Logic and Bit Operations/Compare To Constant  relop=<  const=double(0)  OutDataTypeStr=boolean
  dynamic_shift : ArithShift  BitShiftNumberSource=Input port  BitShiftDirection=Right
      settings: InputPortMap=u0,p1
  dynamic_shift1 : ArithShift  BitShiftNumberSource=Input port  BitShiftDirection=Right
      settings: InputPortMap=u0,p1
  rd_{0..9} (10 alike) : Delay  DelayLength=double(1)  InitialCondition=0  SampleTime=6.25e-09
  xout : Outport  OutDataTypeStr=fixdt(1, 32, 19)  SampleTime=6.25e-09
  yout : Outport  Port=2  OutDataTypeStr=fixdt(1, 32, 19)  SampleTime=6.25e-09
  zout : Outport  Port=3  OutDataTypeStr=fixdt(1, 34, 33)  SampleTime=6.25e-09
  wires:
  MuxX/1 -> xout/1
  MuxY/1 -> yout/1
  rd_4/1 -> MuxX/3
  rd_9/1 -> MuxZ/3
  rd_3/1 -> MuxX/2, MuxY/2, MuxZ/2
  rd_5/1 -> MuxY/1
  MuxZ/1 -> zout/1
  XAdder/1 -> rd_4/1
  XSubtractor/1 -> rd_2/1
  ZSub/1 -> rd_8/1
  yin/1 -> rd_1/1
  xin/1 -> rd_0/1
  rd_1/1 -> compare/1, dynamic_shift1/1, YAdder/1, YSub/1
  rd_6/1 -> MuxY/3
  ZAdder/1 -> rd_9/1
  zin/1 -> rd_7/1
  rd_0/1 -> dynamic_shift/1, XSubtractor/1, XAdder/1
  rd_2/1 -> MuxX/1
  idx/1 -> dynamic_shift/2, dynamic_shift1/2
  YAdder/1 -> rd_5/1
  rd_8/1 -> MuxZ/1
  dynamic_shift/1 -> YAdder/2, YSub/2
  rd_7/1 -> ZSub/1, ZAdder/1
  lut_value/1 -> ZSub/2, ZAdder/2
  compare/1 -> rd_3/1
  dynamic_shift1/1 -> XSubtractor/2, XAdder/2
  YSub/1 -> rd_6/1

== system gm_wlanhdlTimeAndFrequencySynchronization/WLANTimeAndFrequencySynchronization/Coarse CFO Estimation and Correction/Coarse CFO Estimation/Iteration18 ==
  xin : Inport  OutDataTypeStr=fixdt(1, 32, 19)  SampleTime=6.25e-09
  yin : Inport  Port=2  OutDataTypeStr=fixdt(1, 32, 19)  SampleTime=6.25e-09
  zin : Inport  Port=3  OutDataTypeStr=fixdt(1, 34, 33)  SampleTime=6.25e-09
  lut_value : Inport  Port=4  OutDataTypeStr=fixdt(0, 31, 33)  SampleTime=6.25e-09
  idx : Inport  Port=5  OutDataTypeStr=fixdt(0, 6, 0)  SampleTime=6.25e-09
  MuxX : Switch  Criteria=u2 ~= 0  Threshold="fi(0,0,1,0,\"hex\",\"0\")"  OutDataTypeStr=fixdt(1, 32, 19)  SampleTime=6.25e-09  SaturateOnIntegerOverflow=off  InputSameDT=off
  MuxY : Switch  Criteria=u2 ~= 0  Threshold="fi(0,0,1,0,\"hex\",\"0\")"  OutDataTypeStr=fixdt(1, 32, 19)  SampleTime=6.25e-09  SaturateOnIntegerOverflow=off  InputSameDT=off
  MuxZ : Switch  Criteria=u2 ~= 0  Threshold="fi(0,0,1,0,\"hex\",\"0\")"  OutDataTypeStr=fixdt(1, 34, 33)  SampleTime=6.25e-09  SaturateOnIntegerOverflow=off  InputSameDT=off
  XAdder : Sum  OutDataTypeStr=fixdt(1, 32, 19)  SampleTime=6.25e-09
  XSubtractor : Sum  Inputs=+-  OutDataTypeStr=fixdt(1, 32, 19)  AccumDataTypeStr=fixdt(1, 32, 19)  SampleTime=6.25e-09
  YAdder : Sum  OutDataTypeStr=fixdt(1, 32, 19)  SampleTime=6.25e-09
  YSub : Sum  Inputs=+-  OutDataTypeStr=fixdt(1, 32, 19)  AccumDataTypeStr=fixdt(1, 32, 19)  SampleTime=6.25e-09
  ZAdder : Sum  OutDataTypeStr=fixdt(1, 34, 33)  SampleTime=6.25e-09
  ZSub : Sum  Inputs=+-  OutDataTypeStr=fixdt(1, 34, 33)  AccumDataTypeStr=fixdt(1, 34, 33)  SampleTime=6.25e-09
  compare : simulink/Logic and Bit Operations/Compare To Constant  relop=<  const=double(0)  OutDataTypeStr=boolean
  dynamic_shift : ArithShift  BitShiftNumberSource=Input port  BitShiftDirection=Right
      settings: InputPortMap=u0,p1
  dynamic_shift1 : ArithShift  BitShiftNumberSource=Input port  BitShiftDirection=Right
      settings: InputPortMap=u0,p1
  rd_{0..9} (10 alike) : Delay  DelayLength=double(1)  InitialCondition=0  SampleTime=6.25e-09
  xout : Outport  OutDataTypeStr=fixdt(1, 32, 19)  SampleTime=6.25e-09
  yout : Outport  Port=2  OutDataTypeStr=fixdt(1, 32, 19)  SampleTime=6.25e-09
  zout : Outport  Port=3  OutDataTypeStr=fixdt(1, 34, 33)  SampleTime=6.25e-09
  wires:
  MuxY/1 -> yout/1
  rd_4/1 -> MuxX/3
  rd_6/1 -> MuxY/3
  rd_3/1 -> MuxX/2, MuxZ/2, MuxY/2
  rd_5/1 -> MuxY/1
  MuxZ/1 -> zout/1
  rd_9/1 -> MuxZ/3
  rd_8/1 -> MuxZ/1
  XSubtractor/1 -> rd_2/1
  rd_2/1 -> MuxX/1
  YAdder/1 -> rd_5/1
  yin/1 -> rd_1/1
  lut_value/1 -> ZAdder/2, ZSub/2
  zin/1 -> rd_7/1
  ZAdder/1 -> rd_9/1
  MuxX/1 -> xout/1
  rd_1/1 -> compare/1, dynamic_shift1/1, YAdder/1, YSub/1
  rd_7/1 -> ZSub/1, ZAdder/1
  xin/1 -> rd_0/1
  rd_0/1 -> dynamic_shift/1, XSubtractor/1, XAdder/1
  dynamic_shift/1 -> YSub/2, YAdder/2
  XAdder/1 -> rd_4/1
  YSub/1 -> rd_6/1
  idx/1 -> dynamic_shift1/2, dynamic_shift/2
  compare/1 -> rd_3/1
  dynamic_shift1/1 -> XAdder/2, XSubtractor/2
  ZSub/1 -> rd_8/1

== system gm_wlanhdlTimeAndFrequencySynchronization/WLANTimeAndFrequencySynchronization/Coarse CFO Estimation and Correction/Coarse CFO Estimation/Iteration19 ==
  xin : Inport  OutDataTypeStr=fixdt(1, 32, 19)  SampleTime=6.25e-09
  yin : Inport  Port=2  OutDataTypeStr=fixdt(1, 32, 19)  SampleTime=6.25e-09
  zin : Inport  Port=3  OutDataTypeStr=fixdt(1, 34, 33)  SampleTime=6.25e-09
  lut_value : Inport  Port=4  OutDataTypeStr=fixdt(0, 31, 33)  SampleTime=6.25e-09
  idx : Inport  Port=5  OutDataTypeStr=fixdt(0, 6, 0)  SampleTime=6.25e-09
  MuxX : Switch  Criteria=u2 ~= 0  Threshold="fi(0,0,1,0,\"hex\",\"0\")"  OutDataTypeStr=fixdt(1, 32, 19)  SampleTime=6.25e-09  SaturateOnIntegerOverflow=off  InputSameDT=off
  MuxY : Switch  Criteria=u2 ~= 0  Threshold="fi(0,0,1,0,\"hex\",\"0\")"  OutDataTypeStr=fixdt(1, 32, 19)  SampleTime=6.25e-09  SaturateOnIntegerOverflow=off  InputSameDT=off
  MuxZ : Switch  Criteria=u2 ~= 0  Threshold="fi(0,0,1,0,\"hex\",\"0\")"  OutDataTypeStr=fixdt(1, 34, 33)  SampleTime=6.25e-09  SaturateOnIntegerOverflow=off  InputSameDT=off
  XAdder : Sum  OutDataTypeStr=fixdt(1, 32, 19)  SampleTime=6.25e-09
  XSubtractor : Sum  Inputs=+-  OutDataTypeStr=fixdt(1, 32, 19)  AccumDataTypeStr=fixdt(1, 32, 19)  SampleTime=6.25e-09
  YAdder : Sum  OutDataTypeStr=fixdt(1, 32, 19)  SampleTime=6.25e-09
  YSub : Sum  Inputs=+-  OutDataTypeStr=fixdt(1, 32, 19)  AccumDataTypeStr=fixdt(1, 32, 19)  SampleTime=6.25e-09
  ZAdder : Sum  OutDataTypeStr=fixdt(1, 34, 33)  SampleTime=6.25e-09
  ZSub : Sum  Inputs=+-  OutDataTypeStr=fixdt(1, 34, 33)  AccumDataTypeStr=fixdt(1, 34, 33)  SampleTime=6.25e-09
  compare : simulink/Logic and Bit Operations/Compare To Constant  relop=<  const=double(0)  OutDataTypeStr=boolean
  dynamic_shift : ArithShift  BitShiftNumberSource=Input port  BitShiftDirection=Right
      settings: InputPortMap=u0,p1
  dynamic_shift1 : ArithShift  BitShiftNumberSource=Input port  BitShiftDirection=Right
      settings: InputPortMap=u0,p1
  rd_{0..9} (10 alike) : Delay  DelayLength=double(1)  InitialCondition=0  SampleTime=6.25e-09
  xout : Outport  OutDataTypeStr=fixdt(1, 32, 19)  SampleTime=6.25e-09
  yout : Outport  Port=2  OutDataTypeStr=fixdt(1, 32, 19)  SampleTime=6.25e-09
  zout : Outport  Port=3  OutDataTypeStr=fixdt(1, 34, 33)  SampleTime=6.25e-09
  wires:
  MuxX/1 -> xout/1
  MuxY/1 -> yout/1
  MuxZ/1 -> zout/1
  rd_2/1 -> MuxX/1
  rd_6/1 -> MuxY/3
  rd_3/1 -> MuxX/2, MuxZ/2, MuxY/2
  rd_9/1 -> MuxZ/3
  XAdder/1 -> rd_4/1
  YSub/1 -> rd_6/1
  xin/1 -> rd_0/1
  rd_4/1 -> MuxX/3
  yin/1 -> rd_1/1
  dynamic_shift/1 -> YAdder/2, YSub/2
  rd_8/1 -> MuxZ/1
  zin/1 -> rd_7/1
  ZAdder/1 -> rd_9/1
  rd_1/1 -> compare/1, dynamic_shift1/1, YAdder/1, YSub/1
  rd_0/1 -> dynamic_shift/1, XSubtractor/1, XAdder/1
  YAdder/1 -> rd_5/1
  idx/1 -> dynamic_shift/2, dynamic_shift1/2
  XSubtractor/1 -> rd_2/1
  lut_value/1 -> ZSub/2, ZAdder/2
  rd_5/1 -> MuxY/1
  dynamic_shift1/1 -> XSubtractor/2, XAdder/2
  rd_7/1 -> ZSub/1, ZAdder/1
  compare/1 -> rd_3/1
  ZSub/1 -> rd_8/1
